simulink model "sim2_basic"  (R2019b)
settings: Solver=FixedStepAuto  StartTime=0.0  StopTime=60  FixedStep=0.001  RelTol=1e-3
values from neighbouring files (symbols this model uses):
  step_h = 150    [parameters.mat]
undefined symbols (not defined in the file or in its folder): left_wheel_1, left_wheel_2, left_wheel_3, right_wheel_1, right_wheel_2, right_wheel_3, X, Y, Z
libraries: sm_lib x227, nesl_utility x43, autolibmappedmotor x6
(part 4 of 4)

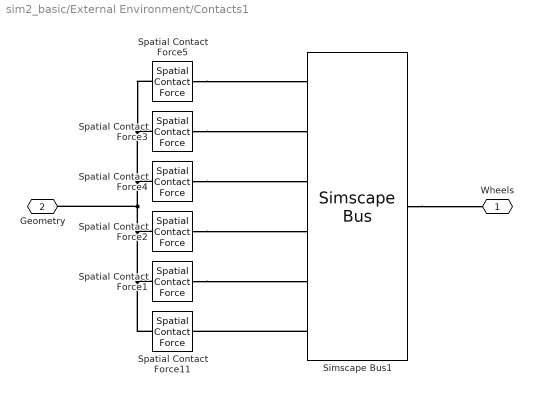
== system sim2_basic/External Environment/Contacts1 ==
  Simscape Bus1 : SimscapeBus  HierarchyStrings=left_wheel_1;left_wheel_2;left_wheel_3;right_wheel_1;right_wheel_2;right_wheel_3
  Spatial Contact Force{1..5,11} (6 alike) : sm_lib/Forces and Torques/Spatial Contact Force  CoefficientOfDynamicFriction=mu_k  CoefficientOfStaticFriction=mu_s  NormalDamping=damping  NormalDampingUnits=N/(m/s)  NormalStiffness=stiffness  NormalStiffnessUnits=N/m  FrictionalCriticalVelocity=v_c  FrictionalCriticalVelocityUnits=m/s  SenseFrictionalForceMagnitude=off  SenseNormalForceMagnitude=off  SenseSeparationDistance=off  NormalTransitionRegionWidth=1e-4  NormalTransitionRegionWidthUnits=m  FrictionType=SmoothStickSlip
      settings: SourceProductName=Simscape Multibody
  Wheels : PMIOPort  Side=Left
  Geometry : PMIOPort  Port=2  Side=Right
  connections:
  Spatial Contact Force3/RConn1 -- Simscape Bus1/LConn2
  Spatial Contact Force4/RConn1 -- Simscape Bus1/LConn3
  Simscape Bus1/LConn6 -- Spatial Contact Force11/RConn1
  Spatial Contact Force1/RConn1 -- Simscape Bus1/LConn5
  Spatial Contact Force2/RConn1 -- Simscape Bus1/LConn4
  Spatial Contact Force5/RConn1 -- Simscape Bus1/LConn1
  Simscape Bus1/RConn1 -- Wheels/RConn1
  Spatial Contact Force3/LConn1 -- Geometry/RConn1 -- Spatial Contact Force11/LConn1 -- Spatial Contact Force1/LConn1 -- Spatial Contact Force2/LConn1 -- Spatial Contact Force4/LConn1 -- Spatial Contact Force5/LConn1

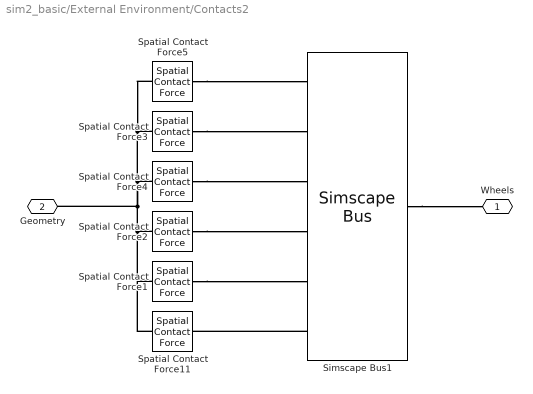
== system sim2_basic/External Environment/Contacts2 ==
  Simscape Bus1 : SimscapeBus  HierarchyStrings=left_wheel_1;left_wheel_2;left_wheel_3;right_wheel_1;right_wheel_2;right_wheel_3
  Spatial Contact Force{1..5,11} (6 alike) : sm_lib/Forces and Torques/Spatial Contact Force  CoefficientOfDynamicFriction=mu_k  CoefficientOfStaticFriction=mu_s  NormalDamping=damping  NormalDampingUnits=N/(m/s)  NormalStiffness=stiffness  NormalStiffnessUnits=N/m  FrictionalCriticalVelocity=v_c  FrictionalCriticalVelocityUnits=m/s  SenseFrictionalForceMagnitude=off  SenseNormalForceMagnitude=off  SenseSeparationDistance=off  NormalTransitionRegionWidth=1e-4  NormalTransitionRegionWidthUnits=m  FrictionType=SmoothStickSlip
      settings: SourceProductName=Simscape Multibody
  Wheels : PMIOPort  Side=Left
  Geometry : PMIOPort  Port=2  Side=Right
  connections:
  Spatial Contact Force4/LConn1 -- Spatial Contact Force2/LConn1 -- Spatial Contact Force1/LConn1 -- Spatial Contact Force11/LConn1 -- Geometry/RConn1 -- Spatial Contact Force3/LConn1 -- Spatial Contact Force5/LConn1
  Simscape Bus1/RConn1 -- Wheels/RConn1
  Spatial Contact Force5/RConn1 -- Simscape Bus1/LConn1
  Spatial Contact Force2/RConn1 -- Simscape Bus1/LConn4
  Spatial Contact Force1/RConn1 -- Simscape Bus1/LConn5
  Simscape Bus1/LConn6 -- Spatial Contact Force11/RConn1
  Spatial Contact Force4/RConn1 -- Simscape Bus1/LConn3
  Spatial Contact Force3/RConn1 -- Simscape Bus1/LConn2

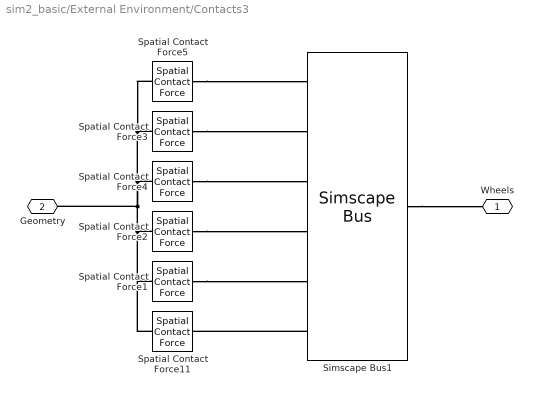
== system sim2_basic/External Environment/Contacts3 ==
  Simscape Bus1 : SimscapeBus  HierarchyStrings=left_wheel_1;left_wheel_2;left_wheel_3;right_wheel_1;right_wheel_2;right_wheel_3
  Spatial Contact Force{1..5,11} (6 alike) : sm_lib/Forces and Torques/Spatial Contact Force  CoefficientOfDynamicFriction=mu_k  CoefficientOfStaticFriction=mu_s  NormalDamping=damping  NormalDampingUnits=N/(m/s)  NormalStiffness=stiffness  NormalStiffnessUnits=N/m  FrictionalCriticalVelocity=v_c  FrictionalCriticalVelocityUnits=m/s  SenseFrictionalForceMagnitude=off  SenseNormalForceMagnitude=off  SenseSeparationDistance=off  NormalTransitionRegionWidth=1e-4  NormalTransitionRegionWidthUnits=m  FrictionType=SmoothStickSlip
      settings: SourceProductName=Simscape Multibody
  Wheels : PMIOPort  Side=Left
  Geometry : PMIOPort  Port=2  Side=Right
  connections:
  Spatial Contact Force5/LConn1 -- Spatial Contact Force4/LConn1 -- Spatial Contact Force2/LConn1 -- Spatial Contact Force1/LConn1 -- Spatial Contact Force11/LConn1 -- Geometry/RConn1 -- Spatial Contact Force3/LConn1
  Simscape Bus1/RConn1 -- Wheels/RConn1
  Spatial Contact Force5/RConn1 -- Simscape Bus1/LConn1
  Spatial Contact Force2/RConn1 -- Simscape Bus1/LConn4
  Spatial Contact Force1/RConn1 -- Simscape Bus1/LConn5
  Simscape Bus1/LConn6 -- Spatial Contact Force11/RConn1
  Spatial Contact Force4/RConn1 -- Simscape Bus1/LConn3
  Spatial Contact Force3/RConn1 -- Simscape Bus1/LConn2

== system sim2_basic/External Environment/Contacts4 ==
  Simscape Bus1 : SimscapeBus  HierarchyStrings=left_wheel_1;left_wheel_2;left_wheel_3;right_wheel_1;right_wheel_2;right_wheel_3
  Spatial Contact Force{1..5,11} (6 alike) : sm_lib/Forces and Torques/Spatial Contact Force  CoefficientOfDynamicFriction=mu_k  CoefficientOfStaticFriction=mu_s  NormalDamping=damping  NormalDampingUnits=N/(m/s)  NormalStiffness=stiffness  NormalStiffnessUnits=N/m  FrictionalCriticalVelocity=v_c  FrictionalCriticalVelocityUnits=m/s  SenseFrictionalForceMagnitude=off  SenseNormalForceMagnitude=off  SenseSeparationDistance=off  NormalTransitionRegionWidth=1e-4  NormalTransitionRegionWidthUnits=m  FrictionType=SmoothStickSlip
      settings: SourceProductName=Simscape Multibody
  Wheels : PMIOPort  Side=Left
  Geometry : PMIOPort  Port=2  Side=Right
  connections:
  Spatial Contact Force3/RConn1 -- Simscape Bus1/LConn2
  Spatial Contact Force4/RConn1 -- Simscape Bus1/LConn3
  Simscape Bus1/LConn6 -- Spatial Contact Force11/RConn1
  Spatial Contact Force1/RConn1 -- Simscape Bus1/LConn5
  Spatial Contact Force2/RConn1 -- Simscape Bus1/LConn4
  Spatial Contact Force5/RConn1 -- Simscape Bus1/LConn1
  Simscape Bus1/RConn1 -- Wheels/RConn1
  Spatial Contact Force3/LConn1 -- Geometry/RConn1 -- Spatial Contact Force11/LConn1 -- Spatial Contact Force1/LConn1 -- Spatial Contact Force2/LConn1 -- Spatial Contact Force4/LConn1 -- Spatial Contact Force5/LConn1

== system sim2_basic/External Environment/Contacts5 ==
  Simscape Bus1 : SimscapeBus  HierarchyStrings=left_wheel_1;left_wheel_2;left_wheel_3;right_wheel_1;right_wheel_2;right_wheel_3
  Spatial Contact Force{1..5,11} (6 alike) : sm_lib/Forces and Torques/Spatial Contact Force  CoefficientOfDynamicFriction=mu_k  CoefficientOfStaticFriction=mu_s  NormalDamping=damping  NormalDampingUnits=N/(m/s)  NormalStiffness=1e6  NormalStiffnessUnits=N/m  FrictionalCriticalVelocity=v_c  FrictionalCriticalVelocityUnits=m/s  SenseFrictionalForceMagnitude=off  SenseNormalForceMagnitude=off  SenseSeparationDistance=off  NormalTransitionRegionWidth=1e-4  NormalTransitionRegionWidthUnits=m  FrictionType=SmoothStickSlip
      settings: SourceProductName=Simscape Multibody
  Wheels : PMIOPort  Side=Left
  Geometry : PMIOPort  Port=2  Side=Right
  connections:
  Spatial Contact Force5/RConn1 -- Simscape Bus1/LConn2
  Spatial Contact Force2/RConn1 -- Simscape Bus1/LConn3
  Simscape Bus1/LConn6 -- Spatial Contact Force11/RConn1
  Spatial Contact Force1/RConn1 -- Simscape Bus1/LConn5
  Spatial Contact Force3/RConn1 -- Simscape Bus1/LConn4
  Spatial Contact Force4/RConn1 -- Simscape Bus1/LConn1
  Simscape Bus1/RConn1 -- Wheels/RConn1
  Spatial Contact Force4/LConn1 -- Spatial Contact Force2/LConn1 -- Geometry/RConn1 -- Spatial Contact Force3/LConn1 -- Spatial Contact Force1/LConn1 -- Spatial Contact Force11/LConn1 -- Spatial Contact Force5/LConn1

== system sim2_basic/External Environment/Contacts6 ==
  Simscape Bus1 : SimscapeBus  HierarchyStrings=left_wheel_1;left_wheel_2;left_wheel_3;right_wheel_1;right_wheel_2;right_wheel_3
  Spatial Contact Force{1..5,11} (6 alike) : sm_lib/Forces and Torques/Spatial Contact Force  CoefficientOfDynamicFriction=mu_k  CoefficientOfStaticFriction=mu_s  NormalDamping=damping  NormalDampingUnits=N/(m/s)  NormalStiffness=1e6  NormalStiffnessUnits=N/m  FrictionalCriticalVelocity=v_c  FrictionalCriticalVelocityUnits=m/s  SenseFrictionalForceMagnitude=off  SenseNormalForceMagnitude=off  SenseSeparationDistance=off  NormalTransitionRegionWidth=1e-4  NormalTransitionRegionWidthUnits=m  FrictionType=SmoothStickSlip
      settings: SourceProductName=Simscape Multibody
  Wheels : PMIOPort  Side=Left
  Geometry : PMIOPort  Port=2  Side=Right
  connections:
  Spatial Contact Force5/RConn1 -- Simscape Bus1/LConn2
  Spatial Contact Force2/RConn1 -- Simscape Bus1/LConn3
  Simscape Bus1/LConn6 -- Spatial Contact Force11/RConn1
  Spatial Contact Force1/RConn1 -- Simscape Bus1/LConn5
  Spatial Contact Force3/RConn1 -- Simscape Bus1/LConn4
  Spatial Contact Force4/RConn1 -- Simscape Bus1/LConn1
  Simscape Bus1/RConn1 -- Wheels/RConn1
  Spatial Contact Force4/LConn1 -- Spatial Contact Force2/LConn1 -- Geometry/RConn1 -- Spatial Contact Force3/LConn1 -- Spatial Contact Force1/LConn1 -- Spatial Contact Force11/LConn1 -- Spatial Contact Force5/LConn1

== system sim2_basic/External Environment/Contacts7 ==
  Simscape Bus1 : SimscapeBus  HierarchyStrings=left_wheel_1;left_wheel_2;left_wheel_3;right_wheel_1;right_wheel_2;right_wheel_3
  Spatial Contact Force{1..5,11} (6 alike) : sm_lib/Forces and Torques/Spatial Contact Force  CoefficientOfDynamicFriction=mu_k  CoefficientOfStaticFriction=mu_s  NormalDamping=damping  NormalDampingUnits=N/(m/s)  NormalStiffness=1e6  NormalStiffnessUnits=N/m  FrictionalCriticalVelocity=v_c  FrictionalCriticalVelocityUnits=m/s  SenseFrictionalForceMagnitude=off  SenseNormalForceMagnitude=off  SenseSeparationDistance=off  NormalTransitionRegionWidth=1e-4  NormalTransitionRegionWidthUnits=m  FrictionType=SmoothStickSlip
      settings: SourceProductName=Simscape Multibody
  Wheels : PMIOPort  Side=Left
  Geometry : PMIOPort  Port=2  Side=Right
  connections:
  Spatial Contact Force5/LConn1 -- Spatial Contact Force11/LConn1 -- Spatial Contact Force1/LConn1 -- Spatial Contact Force3/LConn1 -- Geometry/RConn1 -- Spatial Contact Force2/LConn1 -- Spatial Contact Force4/LConn1
  Simscape Bus1/RConn1 -- Wheels/RConn1
  Spatial Contact Force4/RConn1 -- Simscape Bus1/LConn1
  Spatial Contact Force3/RConn1 -- Simscape Bus1/LConn4
  Spatial Contact Force1/RConn1 -- Simscape Bus1/LConn5
  Simscape Bus1/LConn6 -- Spatial Contact Force11/RConn1
  Spatial Contact Force2/RConn1 -- Simscape Bus1/LConn3
  Spatial Contact Force5/RConn1 -- Simscape Bus1/LConn2

== system sim2_basic/External Environment1/Contacts1 ==
  Simscape Bus1 : SimscapeBus  HierarchyStrings=left_wheel_1;left_wheel_2;left_wheel_3;right_wheel_1;right_wheel_2;right_wheel_3
  Spatial Contact Force{1..5,11} (6 alike) : sm_lib/Forces and Torques/Spatial Contact Force  CoefficientOfDynamicFriction=mu_k  CoefficientOfStaticFriction=mu_s  NormalDamping=damping  NormalDampingUnits=N/(m/s)  NormalStiffness=stiffness  NormalStiffnessUnits=N/m  FrictionalCriticalVelocity=v_c  FrictionalCriticalVelocityUnits=m/s  SenseFrictionalForceMagnitude=off  SenseNormalForceMagnitude=off  SenseSeparationDistance=off  NormalTransitionRegionWidth=1e-4  NormalTransitionRegionWidthUnits=m  FrictionType=SmoothStickSlip
      settings: SourceProductName=Simscape Multibody
  Wheels : PMIOPort  Side=Left
  Geometry : PMIOPort  Port=2  Side=Right
  connections:
  Spatial Contact Force3/RConn1 -- Simscape Bus1/LConn2
  Spatial Contact Force4/RConn1 -- Simscape Bus1/LConn3
  Simscape Bus1/LConn6 -- Spatial Contact Force11/RConn1
  Spatial Contact Force1/RConn1 -- Simscape Bus1/LConn5
  Spatial Contact Force2/RConn1 -- Simscape Bus1/LConn4
  Spatial Contact Force5/RConn1 -- Simscape Bus1/LConn1
  Simscape Bus1/RConn1 -- Wheels/RConn1
  Spatial Contact Force3/LConn1 -- Geometry/RConn1 -- Spatial Contact Force11/LConn1 -- Spatial Contact Force1/LConn1 -- Spatial Contact Force2/LConn1 -- Spatial Contact Force4/LConn1 -- Spatial Contact Force5/LConn1

== system sim2_basic/External Environment1/Contacts10 ==
  Simscape Bus1 : SimscapeBus  HierarchyStrings=left_wheel_1;left_wheel_2;left_wheel_3;right_wheel_1;right_wheel_2;right_wheel_3
  Spatial Contact Force{1..5,11} (6 alike) : sm_lib/Forces and Torques/Spatial Contact Force  CoefficientOfDynamicFriction=mu_k  CoefficientOfStaticFriction=mu_s  NormalDamping=damping  NormalDampingUnits=N/(m/s)  NormalStiffness=stiffness  NormalStiffnessUnits=N/m  FrictionalCriticalVelocity=v_c  FrictionalCriticalVelocityUnits=m/s  SenseFrictionalForceMagnitude=off  SenseNormalForceMagnitude=off  SenseSeparationDistance=off  NormalTransitionRegionWidth=1e-4  NormalTransitionRegionWidthUnits=m  FrictionType=SmoothStickSlip
      settings: SourceProductName=Simscape Multibody
  Wheels : PMIOPort  Side=Left
  Geometry : PMIOPort  Port=2  Side=Right
  connections:
  Spatial Contact Force5/LConn1 -- Spatial Contact Force4/LConn1 -- Spatial Contact Force2/LConn1 -- Spatial Contact Force1/LConn1 -- Spatial Contact Force11/LConn1 -- Geometry/RConn1 -- Spatial Contact Force3/LConn1
  Simscape Bus1/RConn1 -- Wheels/RConn1
  Spatial Contact Force5/RConn1 -- Simscape Bus1/LConn1
  Spatial Contact Force2/RConn1 -- Simscape Bus1/LConn4
  Spatial Contact Force1/RConn1 -- Simscape Bus1/LConn5
  Simscape Bus1/LConn6 -- Spatial Contact Force11/RConn1
  Spatial Contact Force4/RConn1 -- Simscape Bus1/LConn3
  Spatial Contact Force3/RConn1 -- Simscape Bus1/LConn2

== system sim2_basic/External Environment1/Contacts11 ==
  Simscape Bus1 : SimscapeBus  HierarchyStrings=left_wheel_1;left_wheel_2;left_wheel_3;right_wheel_1;right_wheel_2;right_wheel_3
  Spatial Contact Force{1..5,11} (6 alike) : sm_lib/Forces and Torques/Spatial Contact Force  CoefficientOfDynamicFriction=mu_k  CoefficientOfStaticFriction=mu_s  NormalDamping=damping  NormalDampingUnits=N/(m/s)  NormalStiffness=1e6  NormalStiffnessUnits=N/m  FrictionalCriticalVelocity=v_c  FrictionalCriticalVelocityUnits=m/s  SenseFrictionalForceMagnitude=off  SenseNormalForceMagnitude=off  SenseSeparationDistance=off  NormalTransitionRegionWidth=1e-4  NormalTransitionRegionWidthUnits=m  FrictionType=SmoothStickSlip
      settings: SourceProductName=Simscape Multibody
  Wheels : PMIOPort  Side=Left
  Geometry : PMIOPort  Port=2  Side=Right
  connections:
  Spatial Contact Force5/LConn1 -- Spatial Contact Force11/LConn1 -- Spatial Contact Force1/LConn1 -- Spatial Contact Force3/LConn1 -- Geometry/RConn1 -- Spatial Contact Force2/LConn1 -- Spatial Contact Force4/LConn1
  Simscape Bus1/RConn1 -- Wheels/RConn1
  Spatial Contact Force4/RConn1 -- Simscape Bus1/LConn1
  Spatial Contact Force3/RConn1 -- Simscape Bus1/LConn4
  Spatial Contact Force1/RConn1 -- Simscape Bus1/LConn5
  Simscape Bus1/LConn6 -- Spatial Contact Force11/RConn1
  Spatial Contact Force2/RConn1 -- Simscape Bus1/LConn3
  Spatial Contact Force5/RConn1 -- Simscape Bus1/LConn2

== system sim2_basic/External Environment1/Contacts12 ==
  Simscape Bus1 : SimscapeBus  HierarchyStrings=left_wheel_1;left_wheel_2;left_wheel_3;right_wheel_1;right_wheel_2;right_wheel_3
  Spatial Contact Force{1..5,11} (6 alike) : sm_lib/Forces and Torques/Spatial Contact Force  CoefficientOfDynamicFriction=mu_k  CoefficientOfStaticFriction=mu_s  NormalDamping=damping  NormalDampingUnits=N/(m/s)  NormalStiffness=1e6  NormalStiffnessUnits=N/m  FrictionalCriticalVelocity=v_c  FrictionalCriticalVelocityUnits=m/s  SenseFrictionalForceMagnitude=off  SenseNormalForceMagnitude=off  SenseSeparationDistance=off  NormalTransitionRegionWidth=1e-4  NormalTransitionRegionWidthUnits=m  FrictionType=SmoothStickSlip
      settings: SourceProductName=Simscape Multibody
  Wheels : PMIOPort  Side=Left
  Geometry : PMIOPort  Port=2  Side=Right
  connections:
  Spatial Contact Force5/LConn1 -- Spatial Contact Force11/LConn1 -- Spatial Contact Force1/LConn1 -- Spatial Contact Force3/LConn1 -- Geometry/RConn1 -- Spatial Contact Force2/LConn1 -- Spatial Contact Force4/LConn1
  Simscape Bus1/RConn1 -- Wheels/RConn1
  Spatial Contact Force4/RConn1 -- Simscape Bus1/LConn1
  Spatial Contact Force3/RConn1 -- Simscape Bus1/LConn4
  Spatial Contact Force1/RConn1 -- Simscape Bus1/LConn5
  Simscape Bus1/LConn6 -- Spatial Contact Force11/RConn1
  Spatial Contact Force2/RConn1 -- Simscape Bus1/LConn3
  Spatial Contact Force5/RConn1 -- Simscape Bus1/LConn2

== system sim2_basic/External Environment1/Contacts13 ==
  Simscape Bus1 : SimscapeBus  HierarchyStrings=left_wheel_1;left_wheel_2;left_wheel_3;right_wheel_1;right_wheel_2;right_wheel_3
  Spatial Contact Force{1..5,11} (6 alike) : sm_lib/Forces and Torques/Spatial Contact Force  CoefficientOfDynamicFriction=mu_k  CoefficientOfStaticFriction=mu_s  NormalDamping=damping  NormalDampingUnits=N/(m/s)  NormalStiffness=1e6  NormalStiffnessUnits=N/m  FrictionalCriticalVelocity=v_c  FrictionalCriticalVelocityUnits=m/s  SenseFrictionalForceMagnitude=off  SenseNormalForceMagnitude=off  SenseSeparationDistance=off  NormalTransitionRegionWidth=1e-4  NormalTransitionRegionWidthUnits=m  FrictionType=SmoothStickSlip
      settings: SourceProductName=Simscape Multibody
  Wheels : PMIOPort  Side=Left
  Geometry : PMIOPort  Port=2  Side=Right
  connections:
  Spatial Contact Force5/RConn1 -- Simscape Bus1/LConn2
  Spatial Contact Force2/RConn1 -- Simscape Bus1/LConn3
  Simscape Bus1/LConn6 -- Spatial Contact Force11/RConn1
  Spatial Contact Force1/RConn1 -- Simscape Bus1/LConn5
  Spatial Contact Force3/RConn1 -- Simscape Bus1/LConn4
  Spatial Contact Force4/RConn1 -- Simscape Bus1/LConn1
  Simscape Bus1/RConn1 -- Wheels/RConn1
  Spatial Contact Force4/LConn1 -- Spatial Contact Force2/LConn1 -- Geometry/RConn1 -- Spatial Contact Force3/LConn1 -- Spatial Contact Force1/LConn1 -- Spatial Contact Force11/LConn1 -- Spatial Contact Force5/LConn1

== system sim2_basic/External Environment1/Contacts14 ==
  Simscape Bus1 : SimscapeBus  HierarchyStrings=left_wheel_1;left_wheel_2;left_wheel_3;right_wheel_1;right_wheel_2;right_wheel_3
  Spatial Contact Force{1..5,11} (6 alike) : sm_lib/Forces and Torques/Spatial Contact Force  CoefficientOfDynamicFriction=mu_k  CoefficientOfStaticFriction=mu_s  NormalDamping=damping  NormalDampingUnits=N/(m/s)  NormalStiffness=1e6  NormalStiffnessUnits=N/m  FrictionalCriticalVelocity=v_c  FrictionalCriticalVelocityUnits=m/s  SenseFrictionalForceMagnitude=off  SenseNormalForceMagnitude=off  SenseSeparationDistance=off  NormalTransitionRegionWidth=1e-4  NormalTransitionRegionWidthUnits=m  FrictionType=SmoothStickSlip
      settings: SourceProductName=Simscape Multibody
  Wheels : PMIOPort  Side=Left
  Geometry : PMIOPort  Port=2  Side=Right
  connections:
  Spatial Contact Force5/RConn1 -- Simscape Bus1/LConn2
  Spatial Contact Force2/RConn1 -- Simscape Bus1/LConn3
  Simscape Bus1/LConn6 -- Spatial Contact Force11/RConn1
  Spatial Contact Force1/RConn1 -- Simscape Bus1/LConn5
  Spatial Contact Force3/RConn1 -- Simscape Bus1/LConn4
  Spatial Contact Force4/RConn1 -- Simscape Bus1/LConn1
  Simscape Bus1/RConn1 -- Wheels/RConn1
  Spatial Contact Force4/LConn1 -- Spatial Contact Force2/LConn1 -- Geometry/RConn1 -- Spatial Contact Force3/LConn1 -- Spatial Contact Force1/LConn1 -- Spatial Contact Force11/LConn1 -- Spatial Contact Force5/LConn1

== system sim2_basic/External Environment1/Contacts15 ==
  Simscape Bus1 : SimscapeBus  HierarchyStrings=left_wheel_1;left_wheel_2;left_wheel_3;right_wheel_1;right_wheel_2;right_wheel_3
  Spatial Contact Force{1..5,11} (6 alike) : sm_lib/Forces and Torques/Spatial Contact Force  CoefficientOfDynamicFriction=mu_k  CoefficientOfStaticFriction=mu_s  NormalDamping=damping  NormalDampingUnits=N/(m/s)  NormalStiffness=1e6  NormalStiffnessUnits=N/m  FrictionalCriticalVelocity=v_c  FrictionalCriticalVelocityUnits=m/s  SenseFrictionalForceMagnitude=off  SenseNormalForceMagnitude=off  SenseSeparationDistance=off  NormalTransitionRegionWidth=1e-4  NormalTransitionRegionWidthUnits=m  FrictionType=SmoothStickSlip
      settings: SourceProductName=Simscape Multibody
  Wheels : PMIOPort  Side=Left
  Geometry : PMIOPort  Port=2  Side=Right
  connections:
  Spatial Contact Force5/RConn1 -- Simscape Bus1/LConn2
  Spatial Contact Force2/RConn1 -- Simscape Bus1/LConn3
  Simscape Bus1/LConn6 -- Spatial Contact Force11/RConn1
  Spatial Contact Force1/RConn1 -- Simscape Bus1/LConn5
  Spatial Contact Force3/RConn1 -- Simscape Bus1/LConn4
  Spatial Contact Force4/RConn1 -- Simscape Bus1/LConn1
  Simscape Bus1/RConn1 -- Wheels/RConn1
  Spatial Contact Force4/LConn1 -- Spatial Contact Force2/LConn1 -- Geometry/RConn1 -- Spatial Contact Force3/LConn1 -- Spatial Contact Force1/LConn1 -- Spatial Contact Force11/LConn1 -- Spatial Contact Force5/LConn1

== system sim2_basic/External Environment1/Contacts16 ==
  Simscape Bus1 : SimscapeBus  HierarchyStrings=left_wheel_1;left_wheel_2;left_wheel_3;right_wheel_1;right_wheel_2;right_wheel_3
  Spatial Contact Force{1..5,11} (6 alike) : sm_lib/Forces and Torques/Spatial Contact Force  CoefficientOfDynamicFriction=mu_k  CoefficientOfStaticFriction=mu_s  NormalDamping=damping  NormalDampingUnits=N/(m/s)  NormalStiffness=1e6  NormalStiffnessUnits=N/m  FrictionalCriticalVelocity=v_c  FrictionalCriticalVelocityUnits=m/s  SenseFrictionalForceMagnitude=off  SenseNormalForceMagnitude=off  SenseSeparationDistance=off  NormalTransitionRegionWidth=1e-4  NormalTransitionRegionWidthUnits=m  FrictionType=SmoothStickSlip
      settings: SourceProductName=Simscape Multibody
  Wheels : PMIOPort  Side=Left
  Geometry : PMIOPort  Port=2  Side=Right
  connections:
  Spatial Contact Force5/LConn1 -- Spatial Contact Force11/LConn1 -- Spatial Contact Force1/LConn1 -- Spatial Contact Force3/LConn1 -- Geometry/RConn1 -- Spatial Contact Force2/LConn1 -- Spatial Contact Force4/LConn1
  Simscape Bus1/RConn1 -- Wheels/RConn1
  Spatial Contact Force4/RConn1 -- Simscape Bus1/LConn1
  Spatial Contact Force3/RConn1 -- Simscape Bus1/LConn4
  Spatial Contact Force1/RConn1 -- Simscape Bus1/LConn5
  Simscape Bus1/LConn6 -- Spatial Contact Force11/RConn1
  Spatial Contact Force2/RConn1 -- Simscape Bus1/LConn3
  Spatial Contact Force5/RConn1 -- Simscape Bus1/LConn2

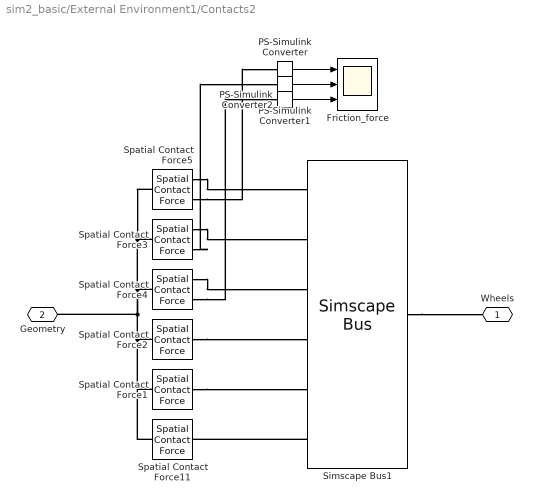
== system sim2_basic/External Environment1/Contacts2 ==
  Friction_force : Scope  NumInputPorts=3
  PS-Simulink Converter : nesl_utility/PS-Simulink Converter  PhysicalDomain=network_engine_domain  SubClassName=ps_output  LeftPortType=input  RightPortType=output  PseudoPeriodic=off  Frequencies=[]  Unit=inherit  AffineConversion=off
  PS-Simulink Converter1 : nesl_utility/PS-Simulink Converter  PhysicalDomain=network_engine_domain  SubClassName=ps_output  LeftPortType=input  RightPortType=output  PseudoPeriodic=off  Frequencies=[]  Unit=inherit  AffineConversion=off
  PS-Simulink Converter2 : nesl_utility/PS-Simulink Converter  PhysicalDomain=network_engine_domain  SubClassName=ps_output  LeftPortType=input  RightPortType=output  PseudoPeriodic=off  Frequencies=[]  Unit=inherit  AffineConversion=off
  Simscape Bus1 : SimscapeBus  HierarchyStrings=left_wheel_1;left_wheel_2;left_wheel_3;right_wheel_1;right_wheel_2;right_wheel_3
  Spatial Contact Force1 : sm_lib/Forces and Torques/Spatial Contact Force  CoefficientOfDynamicFriction=mu_k  CoefficientOfStaticFriction=mu_s  NormalDamping=damping  NormalDampingUnits=N/(m/s)  NormalStiffness=stiffness  NormalStiffnessUnits=N/m  FrictionalCriticalVelocity=v_c  FrictionalCriticalVelocityUnits=m/s  SenseFrictionalForceMagnitude=off  SenseNormalForceMagnitude=off  SenseSeparationDistance=off  NormalTransitionRegionWidth=1e-4  NormalTransitionRegionWidthUnits=m  FrictionType=SmoothStickSlip
      settings: SourceProductName=Simscape Multibody
  Spatial Contact Force11 : sm_lib/Forces and Torques/Spatial Contact Force  CoefficientOfDynamicFriction=mu_k  CoefficientOfStaticFriction=mu_s  NormalDamping=damping  NormalDampingUnits=N/(m/s)  NormalStiffness=stiffness  NormalStiffnessUnits=N/m  FrictionalCriticalVelocity=v_c  FrictionalCriticalVelocityUnits=m/s  SenseFrictionalForceMagnitude=off  SenseNormalForceMagnitude=off  SenseSeparationDistance=off  NormalTransitionRegionWidth=1e-4  NormalTransitionRegionWidthUnits=m  FrictionType=SmoothStickSlip
      settings: SourceProductName=Simscape Multibody
  Spatial Contact Force2 : sm_lib/Forces and Torques/Spatial Contact Force  CoefficientOfDynamicFriction=mu_k  CoefficientOfStaticFriction=mu_s  NormalDamping=damping  NormalDampingUnits=N/(m/s)  NormalStiffness=stiffness  NormalStiffnessUnits=N/m  FrictionalCriticalVelocity=v_c  FrictionalCriticalVelocityUnits=m/s  SenseFrictionalForceMagnitude=off  SenseNormalForceMagnitude=off  SenseSeparationDistance=off  NormalTransitionRegionWidth=1e-4  NormalTransitionRegionWidthUnits=m  FrictionType=SmoothStickSlip
      settings: SourceProductName=Simscape Multibody
  Spatial Contact Force3 : sm_lib/Forces and Torques/Spatial Contact Force  CoefficientOfDynamicFriction=mu_k  CoefficientOfStaticFriction=mu_s  NormalDamping=damping  NormalDampingUnits=N/(m/s)  NormalStiffness=stiffness  NormalStiffnessUnits=N/m  FrictionalCriticalVelocity=v_c  FrictionalCriticalVelocityUnits=m/s  SenseFrictionalForceMagnitude=on  SenseNormalForceMagnitude=off  SenseSeparationDistance=off  NormalTransitionRegionWidth=1e-4  NormalTransitionRegionWidthUnits=m  FrictionType=SmoothStickSlip
      settings: SourceProductName=Simscape Multibody
  Spatial Contact Force4 : sm_lib/Forces and Torques/Spatial Contact Force  CoefficientOfDynamicFriction=mu_k  CoefficientOfStaticFriction=mu_s  NormalDamping=damping  NormalDampingUnits=N/(m/s)  NormalStiffness=stiffness  NormalStiffnessUnits=N/m  FrictionalCriticalVelocity=v_c  FrictionalCriticalVelocityUnits=m/s  SenseFrictionalForceMagnitude=on  SenseNormalForceMagnitude=off  SenseSeparationDistance=off  NormalTransitionRegionWidth=1e-4  NormalTransitionRegionWidthUnits=m  FrictionType=SmoothStickSlip
      settings: SourceProductName=Simscape Multibody
  Spatial Contact Force5 : sm_lib/Forces and Torques/Spatial Contact Force  CoefficientOfDynamicFriction=mu_k  CoefficientOfStaticFriction=mu_s  NormalDamping=damping  NormalDampingUnits=N/(m/s)  NormalStiffness=stiffness  NormalStiffnessUnits=N/m  FrictionalCriticalVelocity=v_c  FrictionalCriticalVelocityUnits=m/s  SenseFrictionalForceMagnitude=on  SenseNormalForceMagnitude=off  SenseSeparationDistance=off  NormalTransitionRegionWidth=1e-4  NormalTransitionRegionWidthUnits=m  FrictionType=SmoothStickSlip
      settings: SourceProductName=Simscape Multibody
  Wheels : PMIOPort  Side=Left
  Geometry : PMIOPort  Port=2  Side=Right
  wires:
  PS-Simulink Converter/1 -> Friction_force/1
  PS-Simulink Converter1/1 -> Friction_force/2
  PS-Simulink Converter2/1 -> Friction_force/3
  connections:
  Spatial Contact Force5/LConn1 -- Spatial Contact Force4/LConn1 -- Spatial Contact Force2/LConn1 -- Spatial Contact Force1/LConn1 -- Spatial Contact Force11/LConn1 -- Geometry/RConn1 -- Spatial Contact Force3/LConn1
  Simscape Bus1/RConn1 -- Wheels/RConn1
  Spatial Contact Force5/RConn1 -- Simscape Bus1/LConn1
  Spatial Contact Force2/RConn1 -- Simscape Bus1/LConn4
  Spatial Contact Force1/RConn1 -- Simscape Bus1/LConn5
  Simscape Bus1/LConn6 -- Spatial Contact Force11/RConn1
  Spatial Contact Force4/RConn1 -- Simscape Bus1/LConn3
  Spatial Contact Force3/RConn1 -- Simscape Bus1/LConn2
  Spatial Contact Force3/RConn2 -- PS-Simulink Converter1/LConn1
  Spatial Contact Force5/RConn2 -- PS-Simulink Converter/LConn1
  Spatial Contact Force4/RConn2 -- PS-Simulink Converter2/LConn1

== system sim2_basic/External Environment1/Contacts3 ==
  Simscape Bus1 : SimscapeBus  HierarchyStrings=left_wheel_1;left_wheel_2;left_wheel_3;right_wheel_1;right_wheel_2;right_wheel_3
  Spatial Contact Force{,1..5} (6 alike) : sm_lib/Forces and Torques/Spatial Contact Force  CoefficientOfDynamicFriction=mu_k  CoefficientOfStaticFriction=mu_s  NormalDamping=damping  NormalDampingUnits=N/(m/s)  NormalStiffness=stiffness  NormalStiffnessUnits=N/m  FrictionalCriticalVelocity=v_c  FrictionalCriticalVelocityUnits=m/s  SenseFrictionalForceMagnitude=off  SenseNormalForceMagnitude=off  SenseSeparationDistance=off  NormalTransitionRegionWidth=1e-4  NormalTransitionRegionWidthUnits=m  FrictionType=SmoothStickSlip
      settings: SourceProductName=Simscape Multibody
  Wheels : PMIOPort  Side=Left
  Ground : PMIOPort  Port=2  Side=Right
  connections:
  Spatial Contact Force5/LConn1 -- Spatial Contact Force4/LConn1 -- Spatial Contact Force2/LConn1 -- Spatial Contact Force1/LConn1 -- Spatial Contact Force/LConn1 -- Ground/RConn1 -- Spatial Contact Force3/LConn1
  Simscape Bus1/RConn1 -- Wheels/RConn1
  Spatial Contact Force5/RConn1 -- Simscape Bus1/LConn1
  Spatial Contact Force2/RConn1 -- Simscape Bus1/LConn4
  Spatial Contact Force1/RConn1 -- Simscape Bus1/LConn5
  Simscape Bus1/LConn6 -- Spatial Contact Force/RConn1
  Spatial Contact Force4/RConn1 -- Simscape Bus1/LConn3
  Spatial Contact Force3/RConn1 -- Simscape Bus1/LConn2

== system sim2_basic/External Environment1/Contacts4 ==
  Simscape Bus1 : SimscapeBus  HierarchyStrings=left_wheel_1;left_wheel_2;left_wheel_3;right_wheel_1;right_wheel_2;right_wheel_3
  Spatial Contact Force{1..5,11} (6 alike) : sm_lib/Forces and Torques/Spatial Contact Force  CoefficientOfDynamicFriction=mu_k  CoefficientOfStaticFriction=mu_s  NormalDamping=damping  NormalDampingUnits=N/(m/s)  NormalStiffness=stiffness  NormalStiffnessUnits=N/m  FrictionalCriticalVelocity=v_c  FrictionalCriticalVelocityUnits=m/s  SenseFrictionalForceMagnitude=off  SenseNormalForceMagnitude=off  SenseSeparationDistance=off  NormalTransitionRegionWidth=1e-4  NormalTransitionRegionWidthUnits=m  FrictionType=SmoothStickSlip
      settings: SourceProductName=Simscape Multibody
  Wheels : PMIOPort  Side=Left
  Geometry : PMIOPort  Port=2  Side=Right
  connections:
  Spatial Contact Force3/RConn1 -- Simscape Bus1/LConn2
  Spatial Contact Force4/RConn1 -- Simscape Bus1/LConn3
  Simscape Bus1/LConn6 -- Spatial Contact Force11/RConn1
  Spatial Contact Force1/RConn1 -- Simscape Bus1/LConn5
  Spatial Contact Force2/RConn1 -- Simscape Bus1/LConn4
  Spatial Contact Force5/RConn1 -- Simscape Bus1/LConn1
  Simscape Bus1/RConn1 -- Wheels/RConn1
  Spatial Contact Force3/LConn1 -- Geometry/RConn1 -- Spatial Contact Force11/LConn1 -- Spatial Contact Force1/LConn1 -- Spatial Contact Force2/LConn1 -- Spatial Contact Force4/LConn1 -- Spatial Contact Force5/LConn1

== system sim2_basic/External Environment1/Contacts5 ==
  Simscape Bus1 : SimscapeBus  HierarchyStrings=left_wheel_1;left_wheel_2;left_wheel_3;right_wheel_1;right_wheel_2;right_wheel_3
  Spatial Contact Force{1..5,11} (6 alike) : sm_lib/Forces and Torques/Spatial Contact Force  CoefficientOfDynamicFriction=mu_k  CoefficientOfStaticFriction=mu_s  NormalDamping=damping  NormalDampingUnits=N/(m/s)  NormalStiffness=1e6  NormalStiffnessUnits=N/m  FrictionalCriticalVelocity=v_c  FrictionalCriticalVelocityUnits=m/s  SenseFrictionalForceMagnitude=off  SenseNormalForceMagnitude=off  SenseSeparationDistance=off  NormalTransitionRegionWidth=1e-4  NormalTransitionRegionWidthUnits=m  FrictionType=SmoothStickSlip
      settings: SourceProductName=Simscape Multibody
  Wheels : PMIOPort  Side=Left
  Geometry : PMIOPort  Port=2  Side=Right
  connections:
  Spatial Contact Force5/RConn1 -- Simscape Bus1/LConn2
  Spatial Contact Force2/RConn1 -- Simscape Bus1/LConn3
  Simscape Bus1/LConn6 -- Spatial Contact Force11/RConn1
  Spatial Contact Force1/RConn1 -- Simscape Bus1/LConn5
  Spatial Contact Force3/RConn1 -- Simscape Bus1/LConn4
  Spatial Contact Force4/RConn1 -- Simscape Bus1/LConn1
  Simscape Bus1/RConn1 -- Wheels/RConn1
  Spatial Contact Force4/LConn1 -- Spatial Contact Force2/LConn1 -- Geometry/RConn1 -- Spatial Contact Force3/LConn1 -- Spatial Contact Force1/LConn1 -- Spatial Contact Force11/LConn1 -- Spatial Contact Force5/LConn1

== system sim2_basic/External Environment1/Contacts6 ==
  Simscape Bus1 : SimscapeBus  HierarchyStrings=left_wheel_1;left_wheel_2;left_wheel_3;right_wheel_1;right_wheel_2;right_wheel_3
  Spatial Contact Force{1..5,11} (6 alike) : sm_lib/Forces and Torques/Spatial Contact Force  CoefficientOfDynamicFriction=mu_k  CoefficientOfStaticFriction=mu_s  NormalDamping=damping  NormalDampingUnits=N/(m/s)  NormalStiffness=1e6  NormalStiffnessUnits=N/m  FrictionalCriticalVelocity=v_c  FrictionalCriticalVelocityUnits=m/s  SenseFrictionalForceMagnitude=off  SenseNormalForceMagnitude=off  SenseSeparationDistance=off  NormalTransitionRegionWidth=1e-4  NormalTransitionRegionWidthUnits=m  FrictionType=SmoothStickSlip
      settings: SourceProductName=Simscape Multibody
  Wheels : PMIOPort  Side=Left
  Geometry : PMIOPort  Port=2  Side=Right
  connections:
  Spatial Contact Force5/RConn1 -- Simscape Bus1/LConn2
  Spatial Contact Force2/RConn1 -- Simscape Bus1/LConn3
  Simscape Bus1/LConn6 -- Spatial Contact Force11/RConn1
  Spatial Contact Force1/RConn1 -- Simscape Bus1/LConn5
  Spatial Contact Force3/RConn1 -- Simscape Bus1/LConn4
  Spatial Contact Force4/RConn1 -- Simscape Bus1/LConn1
  Simscape Bus1/RConn1 -- Wheels/RConn1
  Spatial Contact Force4/LConn1 -- Spatial Contact Force2/LConn1 -- Geometry/RConn1 -- Spatial Contact Force3/LConn1 -- Spatial Contact Force1/LConn1 -- Spatial Contact Force11/LConn1 -- Spatial Contact Force5/LConn1

== system sim2_basic/External Environment1/Contacts7 ==
  Simscape Bus1 : SimscapeBus  HierarchyStrings=left_wheel_1;left_wheel_2;left_wheel_3;right_wheel_1;right_wheel_2;right_wheel_3
  Spatial Contact Force{1..5,11} (6 alike) : sm_lib/Forces and Torques/Spatial Contact Force  CoefficientOfDynamicFriction=mu_k  CoefficientOfStaticFriction=mu_s  NormalDamping=damping  NormalDampingUnits=N/(m/s)  NormalStiffness=1e6  NormalStiffnessUnits=N/m  FrictionalCriticalVelocity=v_c  FrictionalCriticalVelocityUnits=m/s  SenseFrictionalForceMagnitude=off  SenseNormalForceMagnitude=off  SenseSeparationDistance=off  NormalTransitionRegionWidth=1e-4  NormalTransitionRegionWidthUnits=m  FrictionType=SmoothStickSlip
      settings: SourceProductName=Simscape Multibody
  Wheels : PMIOPort  Side=Left
  Geometry : PMIOPort  Port=2  Side=Right
  connections:
  Spatial Contact Force5/LConn1 -- Spatial Contact Force11/LConn1 -- Spatial Contact Force1/LConn1 -- Spatial Contact Force3/LConn1 -- Geometry/RConn1 -- Spatial Contact Force2/LConn1 -- Spatial Contact Force4/LConn1
  Simscape Bus1/RConn1 -- Wheels/RConn1
  Spatial Contact Force4/RConn1 -- Simscape Bus1/LConn1
  Spatial Contact Force3/RConn1 -- Simscape Bus1/LConn4
  Spatial Contact Force1/RConn1 -- Simscape Bus1/LConn5
  Simscape Bus1/LConn6 -- Spatial Contact Force11/RConn1
  Spatial Contact Force2/RConn1 -- Simscape Bus1/LConn3
  Spatial Contact Force5/RConn1 -- Simscape Bus1/LConn2

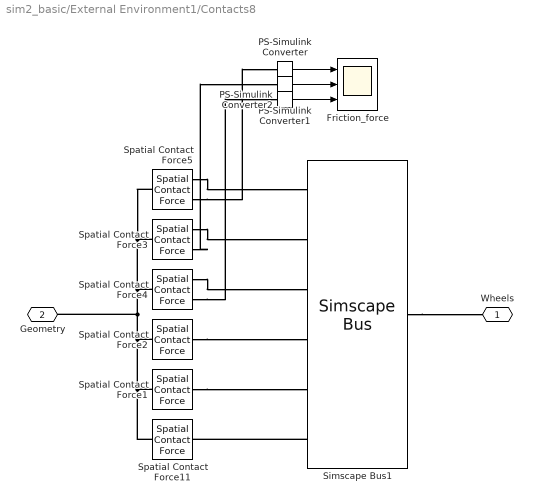
== system sim2_basic/External Environment1/Contacts8 ==
  Friction_force : Scope  NumInputPorts=3
  PS-Simulink Converter : nesl_utility/PS-Simulink Converter  PhysicalDomain=network_engine_domain  SubClassName=ps_output  LeftPortType=input  RightPortType=output  PseudoPeriodic=off  Frequencies=[]  Unit=inherit  AffineConversion=off
  PS-Simulink Converter1 : nesl_utility/PS-Simulink Converter  PhysicalDomain=network_engine_domain  SubClassName=ps_output  LeftPortType=input  RightPortType=output  PseudoPeriodic=off  Frequencies=[]  Unit=inherit  AffineConversion=off
  PS-Simulink Converter2 : nesl_utility/PS-Simulink Converter  PhysicalDomain=network_engine_domain  SubClassName=ps_output  LeftPortType=input  RightPortType=output  PseudoPeriodic=off  Frequencies=[]  Unit=inherit  AffineConversion=off
  Simscape Bus1 : SimscapeBus  HierarchyStrings=left_wheel_1;left_wheel_2;left_wheel_3;right_wheel_1;right_wheel_2;right_wheel_3
  Spatial Contact Force1 : sm_lib/Forces and Torques/Spatial Contact Force  CoefficientOfDynamicFriction=mu_k  CoefficientOfStaticFriction=mu_s  NormalDamping=damping  NormalDampingUnits=N/(m/s)  NormalStiffness=stiffness  NormalStiffnessUnits=N/m  FrictionalCriticalVelocity=v_c  FrictionalCriticalVelocityUnits=m/s  SenseFrictionalForceMagnitude=off  SenseNormalForceMagnitude=off  SenseSeparationDistance=off  NormalTransitionRegionWidth=1e-4  NormalTransitionRegionWidthUnits=m  FrictionType=SmoothStickSlip
      settings: SourceProductName=Simscape Multibody
  Spatial Contact Force11 : sm_lib/Forces and Torques/Spatial Contact Force  CoefficientOfDynamicFriction=mu_k  CoefficientOfStaticFriction=mu_s  NormalDamping=damping  NormalDampingUnits=N/(m/s)  NormalStiffness=stiffness  NormalStiffnessUnits=N/m  FrictionalCriticalVelocity=v_c  FrictionalCriticalVelocityUnits=m/s  SenseFrictionalForceMagnitude=off  SenseNormalForceMagnitude=off  SenseSeparationDistance=off  NormalTransitionRegionWidth=1e-4  NormalTransitionRegionWidthUnits=m  FrictionType=SmoothStickSlip
      settings: SourceProductName=Simscape Multibody
  Spatial Contact Force2 : sm_lib/Forces and Torques/Spatial Contact Force  CoefficientOfDynamicFriction=mu_k  CoefficientOfStaticFriction=mu_s  NormalDamping=damping  NormalDampingUnits=N/(m/s)  NormalStiffness=stiffness  NormalStiffnessUnits=N/m  FrictionalCriticalVelocity=v_c  FrictionalCriticalVelocityUnits=m/s  SenseFrictionalForceMagnitude=off  SenseNormalForceMagnitude=off  SenseSeparationDistance=off  NormalTransitionRegionWidth=1e-4  NormalTransitionRegionWidthUnits=m  FrictionType=SmoothStickSlip
      settings: SourceProductName=Simscape Multibody
  Spatial Contact Force3 : sm_lib/Forces and Torques/Spatial Contact Force  CoefficientOfDynamicFriction=mu_k  CoefficientOfStaticFriction=mu_s  NormalDamping=damping  NormalDampingUnits=N/(m/s)  NormalStiffness=stiffness  NormalStiffnessUnits=N/m  FrictionalCriticalVelocity=v_c  FrictionalCriticalVelocityUnits=m/s  SenseFrictionalForceMagnitude=on  SenseNormalForceMagnitude=off  SenseSeparationDistance=off  NormalTransitionRegionWidth=1e-4  NormalTransitionRegionWidthUnits=m  FrictionType=SmoothStickSlip
      settings: SourceProductName=Simscape Multibody
  Spatial Contact Force4 : sm_lib/Forces and Torques/Spatial Contact Force  CoefficientOfDynamicFriction=mu_k  CoefficientOfStaticFriction=mu_s  NormalDamping=damping  NormalDampingUnits=N/(m/s)  NormalStiffness=stiffness  NormalStiffnessUnits=N/m  FrictionalCriticalVelocity=v_c  FrictionalCriticalVelocityUnits=m/s  SenseFrictionalForceMagnitude=on  SenseNormalForceMagnitude=off  SenseSeparationDistance=off  NormalTransitionRegionWidth=1e-4  NormalTransitionRegionWidthUnits=m  FrictionType=SmoothStickSlip
      settings: SourceProductName=Simscape Multibody
  Spatial Contact Force5 : sm_lib/Forces and Torques/Spatial Contact Force  CoefficientOfDynamicFriction=mu_k  CoefficientOfStaticFriction=mu_s  NormalDamping=damping  NormalDampingUnits=N/(m/s)  NormalStiffness=stiffness  NormalStiffnessUnits=N/m  FrictionalCriticalVelocity=v_c  FrictionalCriticalVelocityUnits=m/s  SenseFrictionalForceMagnitude=on  SenseNormalForceMagnitude=off  SenseSeparationDistance=off  NormalTransitionRegionWidth=1e-4  NormalTransitionRegionWidthUnits=m  FrictionType=SmoothStickSlip
      settings: SourceProductName=Simscape Multibody
  Wheels : PMIOPort  Side=Left
  Geometry : PMIOPort  Port=2  Side=Right
  wires:
  PS-Simulink Converter2/1 -> Friction_force/3
  PS-Simulink Converter1/1 -> Friction_force/2
  PS-Simulink Converter/1 -> Friction_force/1
  connections:
  Spatial Contact Force4/RConn2 -- PS-Simulink Converter2/LConn1
  Spatial Contact Force5/RConn2 -- PS-Simulink Converter/LConn1
  Spatial Contact Force3/RConn2 -- PS-Simulink Converter1/LConn1
  Spatial Contact Force3/RConn1 -- Simscape Bus1/LConn2
  Spatial Contact Force4/RConn1 -- Simscape Bus1/LConn3
  Simscape Bus1/LConn6 -- Spatial Contact Force11/RConn1
  Spatial Contact Force1/RConn1 -- Simscape Bus1/LConn5
  Spatial Contact Force2/RConn1 -- Simscape Bus1/LConn4
  Spatial Contact Force5/RConn1 -- Simscape Bus1/LConn1
  Simscape Bus1/RConn1 -- Wheels/RConn1
  Spatial Contact Force3/LConn1 -- Geometry/RConn1 -- Spatial Contact Force11/LConn1 -- Spatial Contact Force1/LConn1 -- Spatial Contact Force2/LConn1 -- Spatial Contact Force4/LConn1 -- Spatial Contact Force5/LConn1

== system sim2_basic/External Environment1/Contacts9 ==
  Simscape Bus1 : SimscapeBus  HierarchyStrings=left_wheel_1;left_wheel_2;left_wheel_3;right_wheel_1;right_wheel_2;right_wheel_3
  Spatial Contact Force{1..5,11} (6 alike) : sm_lib/Forces and Torques/Spatial Contact Force  CoefficientOfDynamicFriction=mu_k  CoefficientOfStaticFriction=mu_s  NormalDamping=damping  NormalDampingUnits=N/(m/s)  NormalStiffness=stiffness  NormalStiffnessUnits=N/m  FrictionalCriticalVelocity=v_c  FrictionalCriticalVelocityUnits=m/s  SenseFrictionalForceMagnitude=off  SenseNormalForceMagnitude=off  SenseSeparationDistance=off  NormalTransitionRegionWidth=1e-4  NormalTransitionRegionWidthUnits=m  FrictionType=SmoothStickSlip
      settings: SourceProductName=Simscape Multibody
  Wheels : PMIOPort  Side=Left
  Geometry : PMIOPort  Port=2  Side=Right
  connections:
  Spatial Contact Force3/RConn1 -- Simscape Bus1/LConn2
  Spatial Contact Force4/RConn1 -- Simscape Bus1/LConn3
  Simscape Bus1/LConn6 -- Spatial Contact Force11/RConn1
  Spatial Contact Force1/RConn1 -- Simscape Bus1/LConn5
  Spatial Contact Force2/RConn1 -- Simscape Bus1/LConn4
  Spatial Contact Force5/RConn1 -- Simscape Bus1/LConn1
  Simscape Bus1/RConn1 -- Wheels/RConn1
  Spatial Contact Force3/LConn1 -- Geometry/RConn1 -- Spatial Contact Force11/LConn1 -- Spatial Contact Force1/LConn1 -- Spatial Contact Force2/LConn1 -- Spatial Contact Force4/LConn1 -- Spatial Contact Force5/LConn1

== matlab function sim2_basic/Motors1/MATLAB Function ==
  data: u input; y output
function y = fcn(u)
    y = abs(u-0.3)*10+0.5;

== matlab function sim2_basic/Motors/MATLAB Function ==
  data: t input; y1 output; v input; y2 output; y3 output
function [y1, y2, y3] = fcn(t,v)
y1 = 0.25;
y2 = 0.25;
y3 = 0.25;
if t>2.5
    if abs(v) < 0.5
        y1 = 0.25+(12-0.25)*(1-exp(-1*t));
        y2 = 0.25+(8-0.25)*(1-exp(-1*t));
        y3 = 0.25+(10-0.25)*(1-exp(-1*t));
    end
end

== matlab function sim2_basic/Motors1/MATLAB Function1 ==
  data: u input; y output; t input
function y = fcn(u,t)
y = 0;
if abs(u)< 0.075
    y = 0.5;
    if t > 10
        y = 1.4;
        if t > 25
            y = 2;
        end
    end
end
